simulink model "MatlabVentFunction"  (R2020a)
settings: Solver=VariableStepAuto  StartTime=0.0  StopTime=10.0  RelTol=1e-3
settings Model: Creator=Owner  LastModifiedBy=Owner

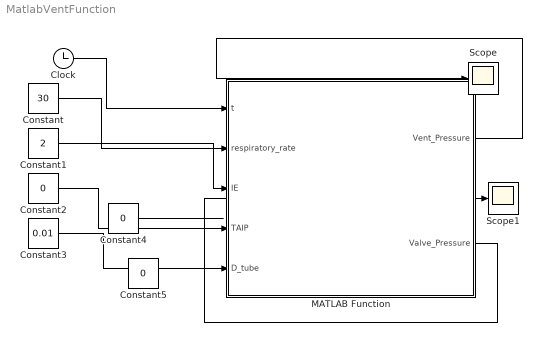
== system MatlabVentFunction ==
  Clock : Clock
  Constant : Constant  Value=30
  Constant1 : Constant  Value=2
  Constant2 : Constant  Value=0
  Constant3 : Constant  Value=0.01
  Constant4 : Constant  Value=0
  Constant5 : Constant  Value=0
  MATLAB Function : MATLAB Function  TreatAsAtomicUnit=on
  Scope : Scope
  Scope1 : Scope
  wires:
  Clock/1 -> MATLAB Function/1(t)
  Constant/1 -> MATLAB Function/2(respiratory_rate)
  Constant1/1 -> MATLAB Function/3(IE)
  Constant2/1 -> MATLAB Function/4(TAIP)
  Constant3/1 -> MATLAB Function/5(D_tube)
  MATLAB Function/1(Vent_Pressure) -> Scope/1
  MATLAB Function/2(Valve_Pressure) -> Scope1/1
  Constant4/1 -> ?

== matlab function MatlabVentFunction/MATLAB Function ==
  data: t input; Vent_Pressure output; respiratory_rate input; IE input; TAIP input; D_tube input; Valve_Pressure output
function [Vent_Pressure,Valve_Pressure] = fcn(t, respiratory_rate, IE, TAIP, D_tube)

%Time Constants
T_Period = 60/respiratory_rate;
T_inspiration = 1/(IE+1) * T_Period;
%T_exhale = T_period - T_inspiration;

cycle_timer = rem(t,T_period);

if TAIP == 0
    if cycle_timer <= T_inspiration
        inhale = 1;
        exhale = 0;
    elseif cycle_timer > T_inspiration
        inhale = 0;
        exhale = 1;
    else
        inhale = 0;
        exhale = 0;
    end
elseif TAIP > 0
    if cycle_timer <= T_inspiration
        if cycle_timer <= TAIP
            slope = input_pressure/TAIP;
            t = cycle_timer - 0;
            inhale = slope*t;
        else
            slope = 1;
            t = cycle_timer - T_inspiration;
            inhale = slope;
        end
    else
        inhale = 0;
        exhale = 1;
    end
else
    inhale = 0;
    exhale = 0;
end
  
MaxValveArea = pi*D_tube^2/4;

Vent_Pressure = inhale*input_pressure;
Valve_Pressure = exhale*MaxValveArea;
